simulink model "TwoMotorModelSimulationX"  (R2020b)
settings: Solver=ode14x  StartTime=0.0  StopTime=SimTime  FixedStep=SimStepTime  RelTol=1e-3
InitFcn:
  | StartupScript
StartFcn:
  | StartupScript
values from neighbouring files (symbols this model uses):
  CF = 372.0    (= 372)    [StartupScript.m]
  Isat = 10.0    (= 10)    [StartupScript.m]
  Ka = 800    [StartupScript.m]
  Kb = 800.0    (= 800)    [StartupScript.m]
  Kda = 1/(Zeroa^2) - Kpa/Polea    (= 0.419912506118)    [StartupScript.m]
  Kdb = 1/(Zerob^2) - Kpb/Poleb    (= 0.414500592554)    [StartupScript.m]
  Kia = 1.0    (= 1)    [StartupScript.m]
  Kib = 1.0    (= 1)    [StartupScript.m]
  Kma = 19.5*1e-3    (= 0.0195)    [StartupScript.m]
  Kmb = 23.4*1e-3    (= 0.0234)    [StartupScript.m]
  Kpa = 2/(Zeroa) - 1/Polea    (= 1.29735721268)    [StartupScript.m]
  Kpb = 2/(Zerob) - 1/Poleb    (= 1.28897849462)    [StartupScript.m]
  PidLim = 1024    [StartupScript.m]
  PidUCGain = 5/1024    (= 0.0048828125)    [StartupScript.m]
  r2d = 180/pi    (= 57.2957795131)    [StartupScript.m]
  sensorGain = 150.0    (= 150)    [StartupScript.m]
  SimStepTime = 1e-3    (= 0.001)    [StartupScript.m]
  Vsat = 18.0    (= 18)    [StartupScript.m]
libraries: cstblocks x6, simulink x1
settings Model: Creator=nisch  LastModifiedBy=nisch

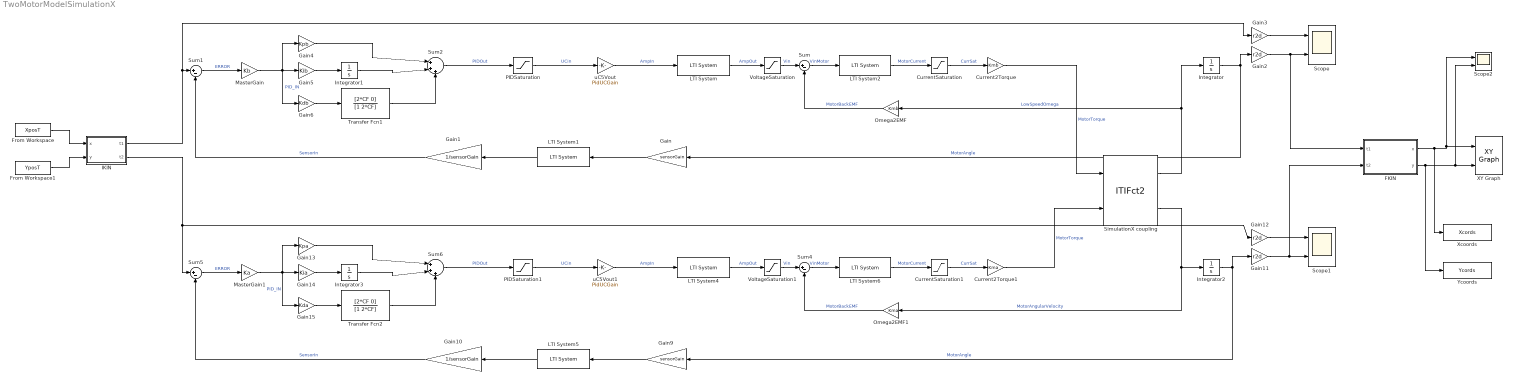
== system TwoMotorModelSimulationX ==
  Current2Torque : Gain  Gain=Kmb
  Current2Torque1 : Gain  Gain=Kma
  CurrentSaturation : Saturate  UpperLimit=Isat  LowerLimit=-Isat
  CurrentSaturation1 : Saturate  UpperLimit=Isat  LowerLimit=-Isat
  FKIN : MATLAB Function  TreatAsAtomicUnit=on
  From Workspace : FromWorkspace  VariableName=XposT
  From Workspace1 : FromWorkspace  VariableName=YposT
  Gain : Gain  Gain=sensorGain
  Gain1 : Gain  Gain=1/sensorGain
  Gain10 : Gain  Gain=1/sensorGain
  Gain{2..3,11..12} (4 alike) : Gain  Gain=r2d
  Gain13 : Gain  Gain=Kpa
  Gain14 : Gain  Gain=Kia
  Gain15 : Gain  Gain=Kda
  Gain4 : Gain  Gain=Kpb
  Gain5 : Gain  Gain=Kib
  Gain6 : Gain  Gain=Kdb
  Gain9 : Gain  Gain=sensorGain
  IKIN : MATLAB Function  TreatAsAtomicUnit=on
  Integrator{,1..3} (4 alike) : Integrator
  LTI System : cstblocks/LTI System  sys=VoltageAmplifier  IC=[]
  LTI System1 : cstblocks/LTI System  sys=Hs  IC=[]
  LTI System2 : cstblocks/LTI System  sys=Electricalb  IC=[]
  LTI System4 : cstblocks/LTI System  sys=VoltageAmplifier  IC=[]
  LTI System5 : cstblocks/LTI System  sys=Hs  IC=[]
  LTI System6 : cstblocks/LTI System  sys=Electricala  IC=[]
  MasterGain : Gain  Gain=Kb
  MasterGain1 : Gain  Gain=Ka
  Omega2EMF : Gain  Gain=Kmb
  Omega2EMF1 : Gain  Gain=Kma
  PIDSaturation : Saturate  UpperLimit=PidLim  LowerLimit=-PidLim
  PIDSaturation1 : Saturate  UpperLimit=PidLim  LowerLimit=-PidLim
  Scope : Scope  NumInputPorts=2
  Scope1 : Scope  NumInputPorts=2
  Scope2 : Scope  NumInputPorts=2
  SimulationX coupling : S-Function  FunctionName=ITIFct2  Parameters=ip, port, ts, nIn, nOut  SFunctionDeploymentMode=off  EnableBusSupport=off  mask{ip='localhost', port=4097, ts=SimStepTime, nIn=2, nOut=2}
      mask prompts: ip "Address: ip"; port "Port Number: port [-]"; ts "Communication Step Size: ts [s]"; nIn "Input Vector Dimension (to SimulationX): nIn [-]"; nOut "Output Vector Dimension (from SimulationX): nOut [-]"
      mask help: Coupling Element
  Sum{,1,4..5} (4 alike) : Sum  Inputs=|+-
  Sum2 : Sum  Inputs=|+++
  Sum6 : Sum  Inputs=|+++
  Transfer Fcn1 : TransferFcn  Numerator=[2*CF 0]  Denominator=[1 2*CF]
  Transfer Fcn2 : TransferFcn  Numerator=[2*CF 0]  Denominator=[1 2*CF]
  VoltageSaturation : Saturate  UpperLimit=Vsat  LowerLimit=-Vsat
  VoltageSaturation1 : Saturate  UpperLimit=Vsat  LowerLimit=-Vsat
  XY Graph : simulink/Sinks/XY Graph  xmin=0  xmax=50  ymin=0  ymax=50  st=-1
  Xcoords : ToWorkspace  VariableName=Xcords  SaveFormat=Timeseries  SampleTime=-1
  Ycoords : ToWorkspace  VariableName=Ycords  SaveFormat=Timeseries  SampleTime=-1
  uC5Vout : Gain  Gain=PidUCGain
  uC5Vout1 : Gain  Gain=PidUCGain
  wires:
  LTI System/1 -> VoltageSaturation/1  "AmpOut"
  PIDSaturation/1 -> uC5Vout/1  "UCin"
  VoltageSaturation/1 -> Sum/1  "Vin"
  IKIN/1(t1) -> Gain3/1, Sum1/1
  uC5Vout/1 -> LTI System/1  "AmpIn"
  Current2Torque/1 -> SimulationX coupling/1  "MotorTorque"
  Gain/1 -> LTI System1/1
  Gain6/1 -> Transfer Fcn1/1
  Gain5/1 -> Integrator1/1
  Sum1/1 -> MasterGain/1  "ERROR"
  LTI System2/1 -> CurrentSaturation/1  "MotorCurrent"
  CurrentSaturation/1 -> Current2Torque/1  "CurrSat"
  Integrator/1 -> Gain/1, Gain2/1  "MotorAngle"
  Gain2/1 -> FKIN/1(t1), Scope/2
  Transfer Fcn1/1 -> Sum2/3
  Sum/1 -> LTI System2/1  "VinMotor"
  Gain4/1 -> Sum2/1
  Integrator1/1 -> Sum2/2
  MasterGain/1 -> Gain6/1, Gain5/1, Gain4/1  "PID_IN"
  Sum2/1 -> PIDSaturation/1  "PIDOut"
  Omega2EMF/1 -> Sum/2  "MotorBackEMF"
  LTI System1/1 -> Gain1/1
  Gain1/1 -> Sum1/2  "SensorIn"
  Gain3/1 -> Scope/1
  Gain9/1 -> LTI System5/1
  Gain11/1 -> Scope1/2, FKIN/2(t2)
  IKIN/2(t2) -> Sum5/1, Gain12/1
  Current2Torque1/1 -> SimulationX coupling/2  "MotorTorque"
  VoltageSaturation1/1 -> Sum4/1  "Vin"
  PIDSaturation1/1 -> uC5Vout1/1  "UCin"
  LTI System5/1 -> Gain10/1
  LTI System4/1 -> VoltageSaturation1/1  "AmpOut"
  SimulationX coupling/2 -> Omega2EMF1/1, Integrator2/1  "MotorAngularVelocity"
  LTI System6/1 -> CurrentSaturation1/1  "MotorCurrent"
  Gain15/1 -> Transfer Fcn2/1
  CurrentSaturation1/1 -> Current2Torque1/1  "CurrSat"
  Gain14/1 -> Integrator3/1
  Omega2EMF1/1 -> Sum4/2  "MotorBackEMF"
  Sum6/1 -> PIDSaturation1/1  "PIDOut"
  MasterGain1/1 -> Gain15/1, Gain14/1, Gain13/1  "PID_IN"
  uC5Vout1/1 -> LTI System4/1  "AmpIn"
  Integrator3/1 -> Sum6/2
  Sum4/1 -> LTI System6/1  "VinMotor"
  Transfer Fcn2/1 -> Sum6/3
  Integrator2/1 -> Gain11/1, Gain9/1  "MotorAngle"
  Gain13/1 -> Sum6/1
  Gain12/1 -> Scope1/1
  Sum5/1 -> MasterGain1/1  "ERROR"
  Gain10/1 -> Sum5/2  "SensorIn"
  FKIN/1(x) -> Xcoords/1, Scope2/1, XY Graph/1
  FKIN/2(y) -> Scope2/2, XY Graph/2, Ycoords/1
  From Workspace/1 -> IKIN/1(x)
  From Workspace1/1 -> IKIN/2(y)
  SimulationX coupling/1 -> Omega2EMF/1, Integrator/1  "LowSpeedOmega"

== matlab function TwoMotorModelSimulationX/IKIN ==
  data: x input; t1 output; y input; t2 output
function [t1, t2] = InverseKin(x, y)
    L1 = 30;
    L2 = 15;
    L3 = sqrt(x^2 + y^2);
    
    a = acos((L1^2 + L3^2 - L2^2)/(2*L1*L3));
    b = acos((L1^2 + L2^2 - L3^2)/(2*L2*L1));
    
    Theta = atan2(y,x);
    
    t1 = real((Theta + a));
    t2 = real(((b - (pi - t1)))); 
end

== matlab function TwoMotorModelSimulationX/FKIN ==
  data: t1 input; x output; t2 input; y output
function [x, y] = ForwardKin(t1, t2)
    
    Larm1 = 30;
    Larm2 = 15;
    
    arm1X = Larm1 * cos(t1*pi/180);
    arm1Y = Larm1 * sin(t1*pi/180);

    arm2X = Larm2 * cos(t2*pi/180) + arm1X;
    arm2Y = Larm2 * sin(t2*pi/180) + arm1Y;
    
    y = arm2Y;
    x = arm2X;
end
